simulink subsystem "Send_Actuator_Cmds"  (R2025a)
settings: Solver=VariableStepAuto  StartTime=0.0  StopTime=10.0  RelTol=1e-3
libraries: px4Peripheralslib x2
settings Model: Creator=gurt1  LastModifiedBy=gurt1

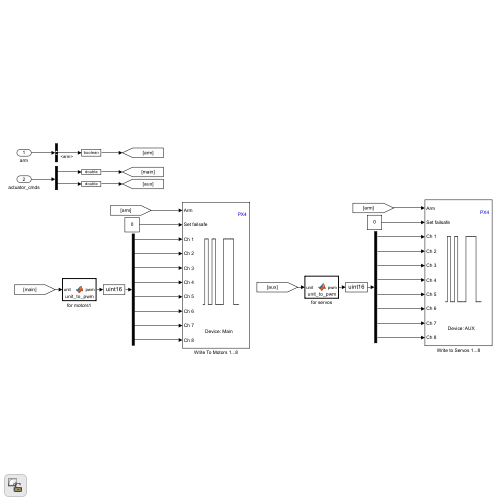
[thumbnail: Simulink's stored preview of the top-level diagram]
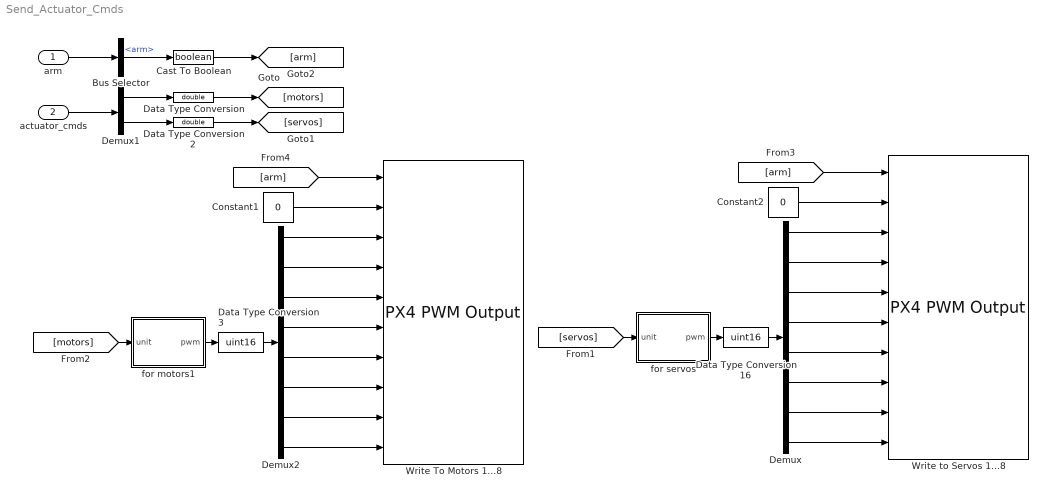
== system Send_Actuator_Cmds ==
  arm : Inport
  actuator_cmds : Inport  Port=2
  Bus Selector : BusSelector  OutputSignals=arm
  Cast To Boolean : DataTypeConversion  OutDataTypeStr=boolean  SaturateOnIntegerOverflow=off  RndMeth=Floor
  Constant1 : Constant  Value=0  OutDataTypeStr=boolean  SampleTime=-1
  Constant2 : Constant  Value=0  OutDataTypeStr=boolean  SampleTime=-1
  Data Type Conversion : DataTypeConversion  OutDataTypeStr=double  SaturateOnIntegerOverflow=off  RndMeth=Floor
  Data Type Conversion16 : DataTypeConversion  OutDataTypeStr=uint16  SaturateOnIntegerOverflow=off  RndMeth=Floor
  Data Type Conversion2 : DataTypeConversion  OutDataTypeStr=double  SaturateOnIntegerOverflow=off  RndMeth=Floor
  Data Type Conversion3 : DataTypeConversion  OutDataTypeStr=uint16  SaturateOnIntegerOverflow=off  RndMeth=Floor
  Demux : Demux  Outputs=8
  Demux1 : Demux  Outputs=[8 8]
  Demux2 : Demux  Outputs=8
  Write To Motors 1...8 : px4Peripheralslib/PX4 PWM Output  pwmDevice=Main  pwmChannel1_=on  pwmChannel2_=on  pwmChannel3_=on  pwmChannel4_=on  pwmChannel5_=on  pwmChannel6_=on  pwmChannel7_=on  pwmChannel8_=on
  Write to Servos 1...8 : px4Peripheralslib/PX4 PWM Output  pwmDevice=AUX  pwmChannel1_=on  pwmChannel2_=on  pwmChannel3_=on  pwmChannel4_=on  pwmChannel5_=on  pwmChannel6_=on  pwmChannel7_=on  pwmChannel8_=on
  for motors1 : MATLAB Function  TreatAsAtomicUnit=on
  for servos : MATLAB Function  TreatAsAtomicUnit=on
  wires:
  for servos/1(pwm) -> Data Type Conversion16/1
  Data Type Conversion2/1 -> [servos]
  [servos] -> for servos/1(unit)
  Constant2/1 -> Write to Servos 1...8/2
  Demux/6 -> Write to Servos 1...8/8
  Demux/2 -> Write to Servos 1...8/4
  Demux/5 -> Write to Servos 1...8/7
  Demux/3 -> Write to Servos 1...8/5
  Demux/4 -> Write to Servos 1...8/6
  Demux/1 -> Write to Servos 1...8/3
  Data Type Conversion/1 -> [motors]
  arm/1 -> Bus Selector/1
  Bus Selector/1 -> Cast To Boolean/1  "<arm>"
  Demux1/1 -> Data Type Conversion/1
  actuator_cmds/1 -> Demux1/1
  Data Type Conversion16/1 -> Demux/1
  [arm] -> Write to Servos 1...8/1
  Demux1/2 -> Data Type Conversion2/1
  Demux/7 -> Write to Servos 1...8/9
  Demux/8 -> Write to Servos 1...8/10
  Cast To Boolean/1 -> [arm]
  Demux2/8 -> Write To Motors 1...8/10
  Demux2/7 -> Write To Motors 1...8/9
  [arm] -> Write To Motors 1...8/1
  Data Type Conversion3/1 -> Demux2/1
  Demux2/1 -> Write To Motors 1...8/3
  Demux2/4 -> Write To Motors 1...8/6
  Demux2/3 -> Write To Motors 1...8/5
  Demux2/5 -> Write To Motors 1...8/7
  Demux2/2 -> Write To Motors 1...8/4
  Demux2/6 -> Write To Motors 1...8/8
  Constant1/1 -> Write To Motors 1...8/2
  [motors] -> for motors1/1(unit)
  for motors1/1(pwm) -> Data Type Conversion3/1

== matlab function Send_Actuator_Cmds/for servos ==
  data: unit input; pwm output
%% unit_to_pwm
% DESCRIPTION: 
%   This function reads in a vector and maps the input from 0 to 1 to the range 
%   of 1000 to 2000. It also checks if any input values are -1 or NaN, and if so, 
%   sets the corresponding output value to 800.
%
% INPUTS: 
%   u   - (Nx1) Input vector with values to be mapped
%
% OUTPUTS:
%   y   - (Nx1) Output vector with mapped PWM values (1000 to 2000 or 800 for invalid inputs)
% 
% WRITTEN BY:
%   Garrett D. Asper
%   Virginia Tech
%   Email: garrettasper@vt.edu
%
% HISTORY:
%   16 SEP 2024 - Created and debugged, GDA
%
% NOMENCLATURE:                                  UNITS:
%   Not Applicable                                  Not Applicable

function pwm = unit_to_pwm(unit)

    % Map the input from 0 to 1 to 1000 to 2000
    unit = (unit+1)./2;
    pwm = unit*1000 + 1000;

    % Iterate through each value to apply constraints
    for i = 1:length(pwm)
        if isnan(unit(i)) || unit(i) == -1
            % Set the output to 800 for invalid inputs (-1 or NaN)
            pwm(i) = 800;
        elseif pwm(i) > 2000
            pwm(i) = 2000;
        elseif pwm(i) < 1000
            pwm(i) = 1000;
        end
    end

end

== matlab function Send_Actuator_Cmds/for motors1 ==
  data: unit input; pwm output
%% unit_to_pwm
% DESCRIPTION: 
%   This function reads in a vector and maps the input from 0 to 1 to the range 
%   of 1000 to 2000. It also checks if any input values are -1 or NaN, and if so, 
%   sets the corresponding output value to 800.
%
% INPUTS: 
%   u   - (Nx1) Input vector with values to be mapped
%
% OUTPUTS:
%   y   - (Nx1) Output vector with mapped PWM values (1000 to 2000 or 800 for invalid inputs)
% 
% WRITTEN BY:
%   Garrett D. Asper
%   Virginia Tech
%   Email: garrettasper@vt.edu
%
% HISTORY:
%   16 SEP 2024 - Created and debugged, GDA
%
% NOMENCLATURE:                                  UNITS:
%   Not Applicable                                  Not Applicable

function pwm = unit_to_pwm(unit)

    % Map the input from 0 to 1 to 1000 to 2000
    pwm = unit*1000 + 1000;

    % Iterate through each value to apply constraints
    for i = 1:length(pwm)
        if isnan(unit(i)) || unit(i) == -1
            % Set the output to 800 for invalid inputs (-1 or NaN)
            pwm(i) = 800;
        elseif pwm(i) > 2000
            pwm(i) = 2000;
        elseif pwm(i) < 1000
            pwm(i) = 1000;
        end
    end

end
